simulink model "ex5"  (R2023b)
settings: Solver=VariableStepAuto  StartTime=0.0  StopTime=10.0  RelTol=1e-3
settings Model: Creator=Andrei  LastModifiedBy=Andrei

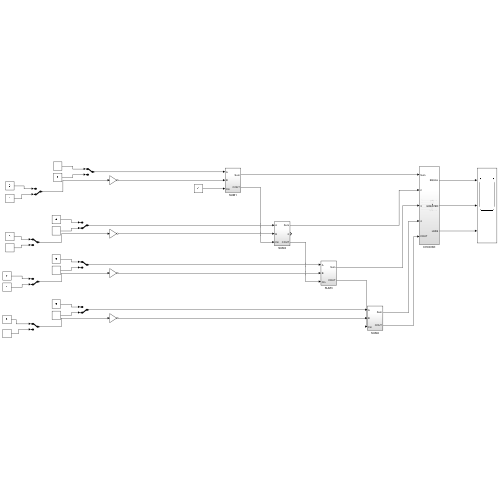
[thumbnail: Simulink's stored preview of the top-level diagram]
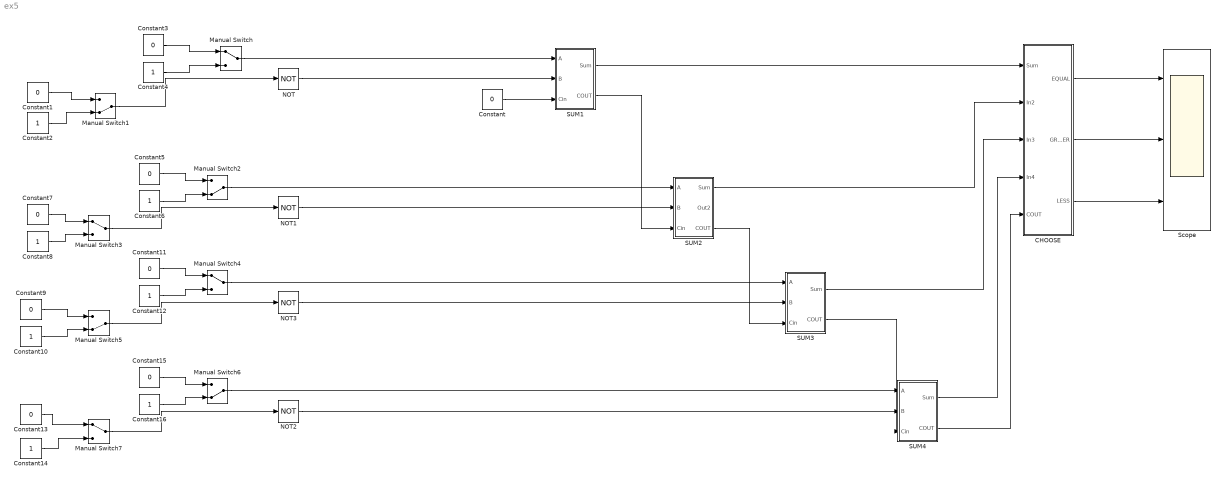
== system ex5 ==
  CHOOSE : Subsystem
  Constant{,1,3,5,7,9,11,13,15} (9 alike) : Constant  Value=0
  Constant{2,4,6,8,10,12,14,16} (8 alike) : Constant
  Manual Switch{,3..4,7} (4 alike) : ManualSwitch
  Manual Switch{1..2,5..6} (4 alike) : ManualSwitch  CurrentSetting=0
  NOT{,1..3} (4 alike) : Logic  Operator=NOT  IconShape=distinctive  AllPortsSameDT=off  OutDataTypeStr=boolean
  SUM1 : Subsystem
  SUM2 : Subsystem
  SUM3 : Subsystem
  SUM4 : Subsystem
  Scope : Scope  NumInputPorts=3
  wires:
  Manual Switch2/1 -> SUM2/1(A)
  Manual Switch6/1 -> SUM4/1(A)
  Constant/1 -> SUM1/3(Cin)
  SUM2/3(COUT) -> SUM3/3(Cin)
  Manual Switch4/1 -> SUM3/1(A)
  SUM3/2(COUT) -> SUM4/3(Cin)
  Manual Switch/1 -> SUM1/1(A)
  SUM1/2(COUT) -> SUM2/3(Cin)
  NOT/1 -> SUM1/2(B)
  NOT1/1 -> SUM2/2(B)
  NOT3/1 -> SUM3/2(B)
  NOT2/1 -> SUM4/2(B)
  SUM4/2(COUT) -> CHOOSE/5(COUT)
  SUM1/1(Sum) -> CHOOSE/1(Sum)
  SUM2/1(Sum) -> CHOOSE/2(In2)
  SUM3/1(Sum) -> CHOOSE/3(In3)
  SUM4/1(Sum) -> CHOOSE/4(In4)
  Manual Switch1/1 -> NOT/1
  Manual Switch3/1 -> NOT1/1
  Manual Switch5/1 -> NOT3/1
  Manual Switch7/1 -> NOT2/1
  Constant1/1 -> Manual Switch1/1
  Constant2/1 -> Manual Switch1/2
  Constant3/1 -> Manual Switch/1
  Constant4/1 -> Manual Switch/2
  Constant5/1 -> Manual Switch2/1
  Constant6/1 -> Manual Switch2/2
  Constant7/1 -> Manual Switch3/1
  Constant8/1 -> Manual Switch3/2
  Constant9/1 -> Manual Switch5/1
  Constant10/1 -> Manual Switch5/2
  Constant11/1 -> Manual Switch4/1
  Constant12/1 -> Manual Switch4/2
  Constant13/1 -> Manual Switch7/1
  Constant14/1 -> Manual Switch7/2
  Constant15/1 -> Manual Switch6/1
  Constant16/1 -> Manual Switch6/2
  CHOOSE/1(EQUAL) -> Scope/1
  CHOOSE/2(GREATER) -> Scope/2
  CHOOSE/3(LESS) -> Scope/3

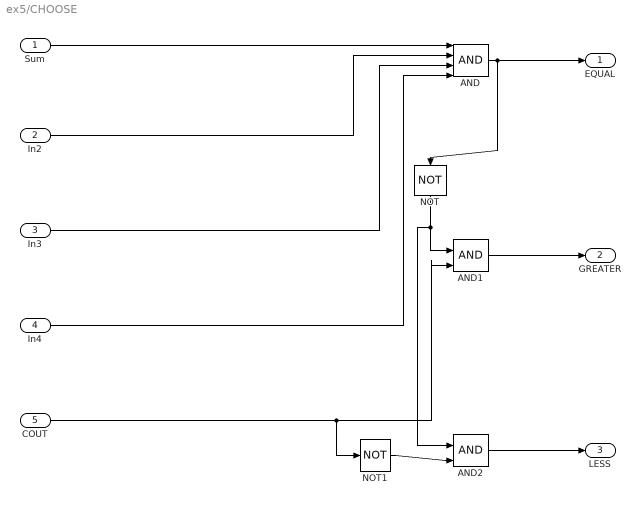
== system ex5/CHOOSE ==
  Sum : Inport
  In2 : Inport  Port=2
  In3 : Inport  Port=3
  In4 : Inport  Port=4
  COUT : Inport  Port=5
  AND : Logic  Inputs=4  IconShape=distinctive  AllPortsSameDT=off  OutDataTypeStr=boolean
  AND1 : Logic  IconShape=distinctive  AllPortsSameDT=off  OutDataTypeStr=boolean
  AND2 : Logic  IconShape=distinctive  AllPortsSameDT=off  OutDataTypeStr=boolean
  NOT : Logic  Operator=NOT  IconShape=distinctive  AllPortsSameDT=off  OutDataTypeStr=boolean
  NOT1 : Logic  Operator=NOT  IconShape=distinctive  AllPortsSameDT=off  OutDataTypeStr=boolean
  EQUAL : Outport
  GREATER : Outport  Port=2
  LESS : Outport  Port=3
  wires:
  AND/1 -> NOT/1, EQUAL/1
  In4/1 -> AND/4
  In3/1 -> AND/3
  In2/1 -> AND/2
  Sum/1 -> AND/1
  COUT/1 -> AND1/2, NOT1/1
  AND1/1 -> GREATER/1
  NOT/1 -> AND2/1, AND1/1
  NOT1/1 -> AND2/2
  AND2/1 -> LESS/1

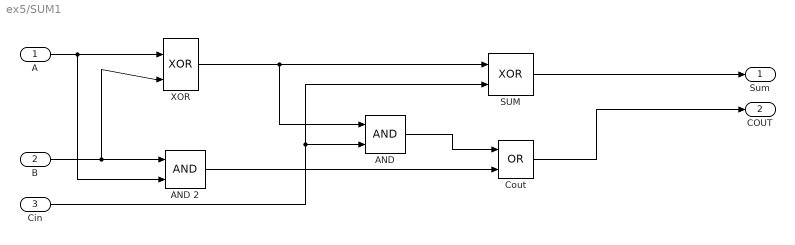
== system ex5/SUM1 ==
  A : Inport
  B : Inport  Port=2
  Cin : Inport  Port=3
  AND : Logic  IconShape=distinctive  AllPortsSameDT=off  OutDataTypeStr=boolean
  "AND 2 " : Logic  IconShape=distinctive  AllPortsSameDT=off  OutDataTypeStr=boolean
  Cout : Logic  Operator=OR  IconShape=distinctive  AllPortsSameDT=off  OutDataTypeStr=boolean
  SUM : Logic  Operator=XOR  IconShape=distinctive  AllPortsSameDT=off  OutDataTypeStr=boolean
  XOR : Logic  Operator=XOR  IconShape=distinctive  AllPortsSameDT=off  OutDataTypeStr=boolean
  Sum : Outport
  COUT : Outport  Port=2
  wires:
  XOR/1 -> SUM/1, AND/1
  SUM/1 -> Sum/1
  AND/1 -> Cout/1
  "AND 2 "/1 -> Cout/2
  Cout/1 -> COUT/1
  Cin/1 -> SUM/2, AND/2
  B/1 -> XOR/2, "AND 2 "/1
  A/1 -> XOR/1, "AND 2 "/2

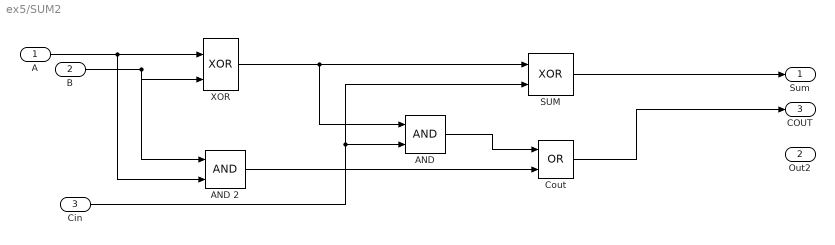
== system ex5/SUM2 ==
  A : Inport
  B : Inport  Port=2
  Cin : Inport  Port=3
  AND : Logic  IconShape=distinctive  AllPortsSameDT=off  OutDataTypeStr=boolean
  "AND 2 " : Logic  IconShape=distinctive  AllPortsSameDT=off  OutDataTypeStr=boolean
  Cout : Logic  Operator=OR  IconShape=distinctive  AllPortsSameDT=off  OutDataTypeStr=boolean
  SUM : Logic  Operator=XOR  IconShape=distinctive  AllPortsSameDT=off  OutDataTypeStr=boolean
  XOR : Logic  Operator=XOR  IconShape=distinctive  AllPortsSameDT=off  OutDataTypeStr=boolean
  Sum : Outport
  Out2 : Outport  Port=2
  COUT : Outport  Port=3
  wires:
  XOR/1 -> SUM/1, AND/1
  SUM/1 -> Sum/1
  AND/1 -> Cout/1
  "AND 2 "/1 -> Cout/2
  Cout/1 -> COUT/1
  Cin/1 -> SUM/2, AND/2
  B/1 -> XOR/2, "AND 2 "/1
  A/1 -> XOR/1, "AND 2 "/2

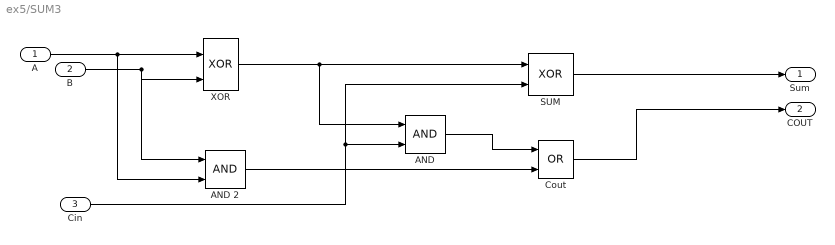
== system ex5/SUM3 ==
  A : Inport
  B : Inport  Port=2
  Cin : Inport  Port=3
  AND : Logic  IconShape=distinctive  AllPortsSameDT=off  OutDataTypeStr=boolean
  "AND 2 " : Logic  IconShape=distinctive  AllPortsSameDT=off  OutDataTypeStr=boolean
  Cout : Logic  Operator=OR  IconShape=distinctive  AllPortsSameDT=off  OutDataTypeStr=boolean
  SUM : Logic  Operator=XOR  IconShape=distinctive  AllPortsSameDT=off  OutDataTypeStr=boolean
  XOR : Logic  Operator=XOR  IconShape=distinctive  AllPortsSameDT=off  OutDataTypeStr=boolean
  Sum : Outport
  COUT : Outport  Port=2
  wires:
  XOR/1 -> SUM/1, AND/1
  SUM/1 -> Sum/1
  AND/1 -> Cout/1
  "AND 2 "/1 -> Cout/2
  Cout/1 -> COUT/1
  Cin/1 -> SUM/2, AND/2
  B/1 -> XOR/2, "AND 2 "/1
  A/1 -> XOR/1, "AND 2 "/2

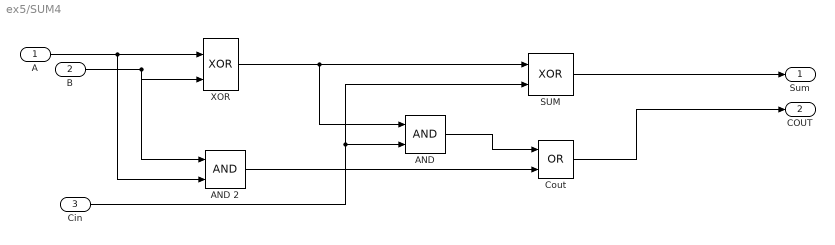
== system ex5/SUM4 ==
  A : Inport
  B : Inport  Port=2
  Cin : Inport  Port=3
  AND : Logic  IconShape=distinctive  AllPortsSameDT=off  OutDataTypeStr=boolean
  "AND 2 " : Logic  IconShape=distinctive  AllPortsSameDT=off  OutDataTypeStr=boolean
  Cout : Logic  Operator=OR  IconShape=distinctive  AllPortsSameDT=off  OutDataTypeStr=boolean
  SUM : Logic  Operator=XOR  IconShape=distinctive  AllPortsSameDT=off  OutDataTypeStr=boolean
  XOR : Logic  Operator=XOR  IconShape=distinctive  AllPortsSameDT=off  OutDataTypeStr=boolean
  Sum : Outport
  COUT : Outport  Port=2
  wires:
  XOR/1 -> SUM/1, AND/1
  SUM/1 -> Sum/1
  AND/1 -> Cout/1
  "AND 2 "/1 -> Cout/2
  Cout/1 -> COUT/1
  Cin/1 -> SUM/2, AND/2
  B/1 -> XOR/2, "AND 2 "/1
  A/1 -> XOR/1, "AND 2 "/2
